simulink model "tut1"  (Simulink 7.0)
settings: Solver=ode45  StartTime=0.0  StopTime=10.0  RelTol=1e-3
libraries: xbsIndex_r4 x7, xps_library x7
settings Model: Creator=user  LastModifiedBy=user

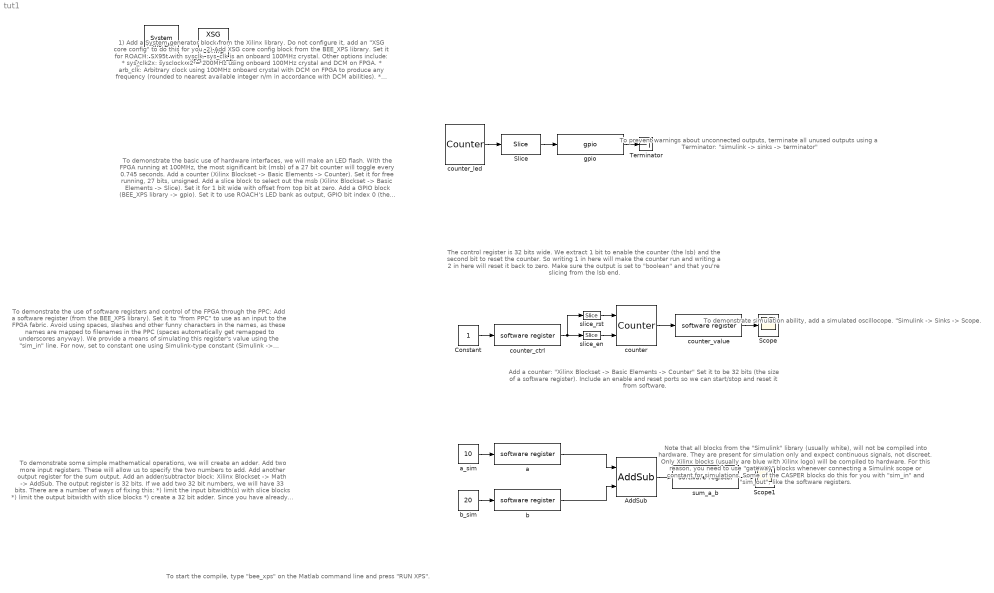
== system tut1 ==
  note: 1) Add a System generator block from the Xilinx library. Do not configure it, add an "XSG core config" to do this for you.
      | 2) Add XSG core config block from the BEE_XPS library. Set it for ROACH: SX95t with sysclk. sys_clk is an onboard 100MHz crystal. Other options include:
      | * sys_clk2x: sysclock x2 = 200MHz using onboard 100MHz crystal and DCM on FPGA.
      | * arb_clk: Arbitrary clock using 100MHz onboard crystal with DCM on FPGA to produce any frequency (rounded to nearest available integer n/m in accordance with DCM abilities).
      | * aux_clk (usr_clk on older platforms): SMA input to board. PLL'd versions of these clocks are also available.
      | * adcX_clk: For use in conjuction with ADC boards, clock the FPGA off the ADC. For iADC and KATADC, this is 1/4 of sampling rate (ADCs demux internally). You need to use one of these clocks if you are using an ADC.
  note: To demonstrate the use of software registers and control of the FPGA through the PPC:
      |
      | Add a software register (from the BEE_XPS library).
      | Set it to "from PPC" to use as an input to the FPGA fabric.
      | Avoid using spaces, slashes and other funny characters in the names,
      | as these names are mapped to filenames in the PPC
      | (spaces automatically get remapped to underscores anyway).
      |
      | We provide a means of simulating this register's value using the "sim_in" line.
      | For now, set to constant one using Simulink-type constant (Simulink -> sources -> constant).
      |
      | Add a second register for the counter output to "To PPC". Give it a useful name.
  note: Add a counter: "Xilinx Blockset -> Basic Elements -> Counter"
      | Set it to be 32 bits (the size of a software register).
      | Include an enable and reset ports so we can start/stop and reset it from software.
  note: To prevent warnings about unconnected outputs,
      | terminate all unused outputs using a Terminator:
      | "simulink -> sinks -> terminator"
  note: The control register is 32 bits wide.
      | We extract 1 bit to enable the counter (the lsb)
      | and the second bit to reset the counter.
      |
      | So writing 1 in here will make the counter run
      | and writing a 2 in here will reset it back to zero.
      |
      | Make sure the output is set to "boolean" and
      | that you're slicing from the lsb end.
  note: To demonstrate simulation ability,
      | add a simulated oscillocope.
      | "Simulink -> Sinks -> Scope.
  note: Note that all blocks from the "Simulink" library (usually white),
      | will not be compiled into hardware. They are present for simulation only
      | and expect continuous signals, not discreet.
      |
      | Only Xilinx blocks (usually are blue with Xilinx logo)
      | will be compiled to hardware.
      |
      | For this reason, you need to use "gateway" blocks whenever
      | connecting a Simulink scope or constant for simulations.
      | Some of the CASPER blocks do this for you with "sim_in"
      | and "sim_out", like the software registers.
  note: To demonstrate the basic use of hardware interfaces,
      | we will make an LED flash.
      |
      | With the FPGA running at 100MHz, the most significant bit (msb)
      | of a 27 bit counter will toggle every 0.745 seconds.
      |
      | Add a counter (Xilinx Blockset -> Basic Elements -> Counter).
      | Set it for free running, 27 bits, unsigned.
      |
      | Add a slice block to select out the msb
      | (Xilinx Blockset -> Basic Elements -> Slice).
      | Set it for 1 bit wide with offset from top bit at zero.
      |
      | Add a GPIO block (BEE_XPS library -> gpio).
      | Set it to use ROACH's LED bank as output,
      | GPIO bit index 0 (the first LED).
  note: To demonstrate some simple mathematical operations, we will create an adder.
      |
      | Add two more input registers. These will allow us to specify the two numbers to add.
      | Add another output register for the sum output.
      |
      | Add an adder/subtractor block: Xilinx Blockset -> Math -> AddSub.
      | The output register is 32 bits. If we add two 32 bit numbers, we will have 33 bits.
      | There are a number of ways of fixing this:
      |  *) limit the input bitwidth(s) with slice blocks
      |  *) limit the output bitwidth with slice blocks
      |  *) create a 32 bit adder.
      | Since you have already seen slice blocks demonstrated, let's try to set the AddSub block to
      | be a 32 bit saturating adder. On the second tab, set it for user-defined precision, unsigned 32 bits.
      | Under overflow, set it to saturate. Now if we add two very large numbers, it will simply return 2^32 -1.
  note: To start the compile, type "bee_xps" on the Matlab command line and press "RUN XPS".
  " System Generator" : xbsIndex_r4/ System Generator  Tag=genX  SystemSampleTime=-1  xilinxfamily=virtex5  part=xc5vsx95t  speed=-1  package=ff1136  synthesis_tool=XST  clock_wrapper=Clock Enables  directory=./tut1/sysgen  testbench=off  simulink_period=1  sysclk_period=10  dcm_input_clock_period=100  incr_netlist=off  trim_vbits=Everywhere in SubSystem  dbl_ovrd=According to Block Masks  core_generation=According to Block Masks  run_coregen=off  deprecated_control=off  eval_field=0  block_type=sysgen
      settings: block_version=10.1.3
  AddSub : xbsIndex_r4/AddSub  mode=Addition  use_carryin=off  use_carryout=off  en=off  latency=0  precision=User Defined  arith_type=Unsigned  n_bits=32  bin_pt=0  quantization=Truncate  overflow=Saturate  dbl_ovrd=off  use_behavioral_HDL=off  pipelined=off  use_rpm=on  hw_selection=Fabric  block_type=addsub
      settings: block_version=10.1.3
  Constant : Constant  OutDataType=sfix(16)  OutScaling=2^0
  Scope : Scope
  Scope1 : Scope
  Slice : xbsIndex_r4/Slice  nbits=1  boolean_output=off  mode=Upper Bit Location + Width  bit1=0  base1=MSB of Input  bit0=0  base0=LSB of Input  dbl_ovrd=off  block_type=slice
      settings: infoedit="Extracts a given range of bits from each input sample and presents it at the output.  The output type is ordinarily unsigned with binary point at zero, but can be Boolean when the slice is one bit wide.<P><P>Hardware notes: In hardware this block costs nothing."  block_version=10.1.3
  Terminator : Terminator
  XSG core config : xps_library/XSG core config  Tag=xps:xsg  SystemSampleTime=-1  hw_sys=ROACH:sx95t  ibob_linux=off  clk_src=sys_clk  iBOB_clk_src=sys_clk  BEE2_ctrl_clk_src=sys_clk  BEE2_usr_clk_src=sys_clk  ROACH_clk_src=sys_clk  CORR_clk_src=sys_clk  gpio_clk_io_group=iBOB:sma  gpio_clk_bit_index=0  clk_rate=100  sample_period=1  synthesis_tool=XST  mpc_type=powerpc440_ext
  a : xps_library/software register  Tag=xps:sw_reg  SystemSampleTime=-1  io_dir=From Processor  arith_type=Unsigned  bitwidth=32  bin_pt=0  sample_period=1  gw_name=tut1_a_user_data_out
      link override tut1_a_user_data_out: arith_type=Unsigned  n_bits=32  bin_pt=0  period=1
  a_sim : Constant  Value=10  OutDataType=sfix(16)  OutScaling=2^0
  b : xps_library/software register  Tag=xps:sw_reg  SystemSampleTime=-1  io_dir=From Processor  arith_type=Unsigned  bitwidth=32  bin_pt=0  sample_period=1  gw_name=tut1_b_user_data_out
      link override tut1_b_user_data_out: arith_type=Unsigned  n_bits=32  bin_pt=0  period=1
  b_sim : Constant  Value=20  OutDataType=sfix(16)  OutScaling=2^0
  counter : xbsIndex_r4/Counter  cnt_type=Free Running  cnt_to=Inf  operation=Up  start_count=0  cnt_by_val=1  arith_type=Unsigned  n_bits=32  bin_pt=0  load_pin=off  rst=on  en=on  explicit_period=on  period=1  dbl_ovrd=off  use_behavioral_HDL=off  use_rpm=off  implementation=Fabric  block_type=counter
  counter_ctrl : xps_library/software register  Tag=xps:sw_reg  SystemSampleTime=-1  io_dir=From Processor  arith_type=Unsigned  bitwidth=32  bin_pt=0  sample_period=1  gw_name=tut1_counter_ctrl_user_data_out
      link override tut1_counter_ctrl_user_data_out: arith_type=Unsigned  n_bits=32  bin_pt=0  period=1
  counter_led : xbsIndex_r4/Counter  cnt_type=Free Running  cnt_to=Inf  operation=Up  start_count=0  cnt_by_val=1  arith_type=Unsigned  n_bits=27  bin_pt=0  load_pin=off  rst=off  en=off  explicit_period=on  period=1  dbl_ovrd=off  use_behavioral_HDL=off  use_rpm=off  implementation=Fabric  block_type=counter
  counter_value : xps_library/software register  Tag=xps:sw_reg  SystemSampleTime=-1  io_dir=To Processor  arith_type=Unsigned  bitwidth=32  bin_pt=0  sample_period=1  gw_name=tut1_counter_value_user_data_in
      link override convert: arith_type=Unsigned  n_bits=32  bin_pt=0
  gpio : xps_library/gpio  Tag=xps:gpio  SystemSampleTime=-1  io_group=ROACH:led  io_dir=out  arith_type=Boolean  bitwidth=1  bin_pt=0  bit_index=0  sample_period=1  use_single_ended=off  use_ddr=off  reg_iob=on  reg_clk_phase=0  termination=None
      link override convert: arith_type=Boolean  n_bits=1  bin_pt=0
  slice_en : xbsIndex_r4/Slice  nbits=1  boolean_output=on  mode=Lower Bit Location + Width  bit1=0  base1=MSB of Input  bit0=0  base0=LSB of Input  dbl_ovrd=off  block_type=slice
      settings: infoedit="Extracts a given range of bits from each input sample and presents it at the output.  The output type is ordinarily unsigned with binary point at zero, but can be Boolean when the slice is one bit wide.<P><P>Hardware notes: In hardware this block costs nothing."  block_version=10.1.3
  slice_rst : xbsIndex_r4/Slice  nbits=1  boolean_output=on  mode=Lower Bit Location + Width  bit1=0  base1=MSB of Input  bit0=1  base0=LSB of Input  dbl_ovrd=off  block_type=slice
      settings: infoedit="Extracts a given range of bits from each input sample and presents it at the output.  The output type is ordinarily unsigned with binary point at zero, but can be Boolean when the slice is one bit wide.<P><P>Hardware notes: In hardware this block costs nothing."  block_version=10.1.3
  sum_a_b : xps_library/software register  Tag=xps:sw_reg  SystemSampleTime=-1  io_dir=To Processor  arith_type=Unsigned  bitwidth=32  bin_pt=0  sample_period=1  gw_name=tut1_sum_a_b_user_data_in
      link override convert: arith_type=Unsigned  n_bits=32  bin_pt=0
  wires:
  Constant/1 -> counter_ctrl/1
  counter_ctrl/1 -> slice_en/1, slice_rst/1
  slice_rst/1 -> counter/1
  slice_en/1 -> counter/2
  counter/1 -> counter_value/1
  counter_value/1 -> Scope/1
  counter_led/1 -> Slice/1
  Slice/1 -> gpio/1
  gpio/1 -> Terminator/1
  a_sim/1 -> a/1
  b_sim/1 -> b/1
  a/1 -> AddSub/1
  b/1 -> AddSub/2
  sum_a_b/1 -> Scope1/1
  AddSub/1 -> sum_a_b/1
